simulink model "task_3_scheme"  (R2024a)
settings: Solver=VariableStepAuto  StartTime=0.0  StopTime=10.0  RelTol=1e-3
settings Model: Creator=alexe  LastModifiedBy=alexe

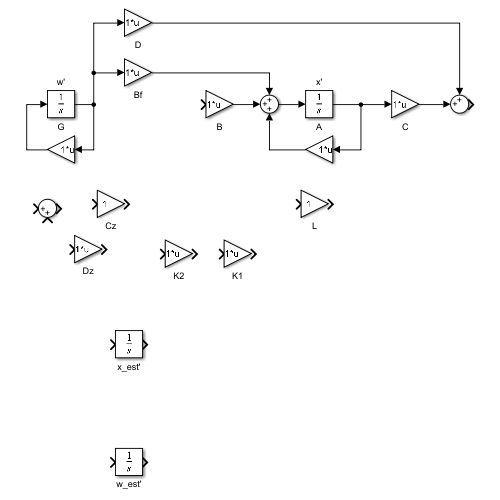
[thumbnail: Simulink's stored preview of the top-level diagram]
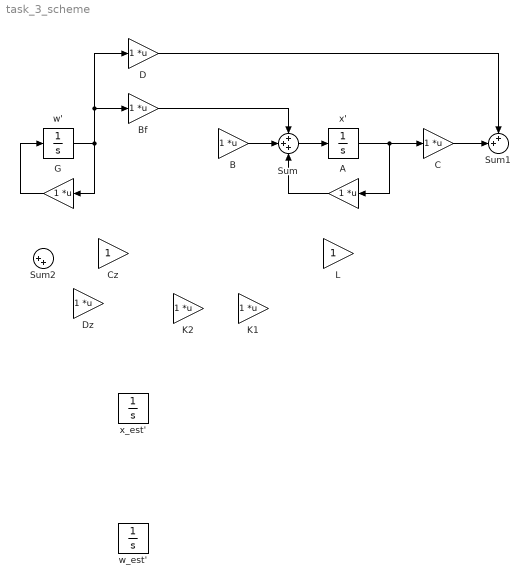
== system task_3_scheme ==
  A : Gain  Multiplication=Matrix(K*u)
  B : Gain  Multiplication=Matrix(K*u)
  Bf : Gain  Multiplication=Matrix(K*u)
  C : Gain  Multiplication=Matrix(K*u)
  Cz : Gain
  D : Gain  Multiplication=Matrix(K*u)
  Dz : Gain  Multiplication=Matrix(K*u)
  G : Gain  Multiplication=Matrix(K*u)
  K1 : Gain  Multiplication=Matrix(K*u)
  K2 : Gain  Multiplication=Matrix(K*u)
  L : Gain
  Sum : Sum  Inputs=+++
  Sum1 : Sum  Inputs=++|
  Sum2 : Sum  Inputs=|++
  w' : Integrator  InitialCondition=[1;1;1;1]
  w_est' : Integrator
  x' : Integrator  InitialCondition=[0;0;0]
  x_est' : Integrator
  wires:
  x'/1 -> A/1, C/1
  Sum/1 -> x'/1
  w'/1 -> D/1, Bf/1, G/1
  G/1 -> w'/1
  A/1 -> Sum/3
  B/1 -> Sum/2
  Bf/1 -> Sum/1
  D/1 -> Sum1/1
  C/1 -> Sum1/2
